simulink subsystem "Segway"  (R2023a)
settings: Solver=VariableStepAuto  StartTime=0.0  StopTime=10.0  RelTol=1e-3
settings Model: Creator=mfilo  LastModifiedBy=mfilo

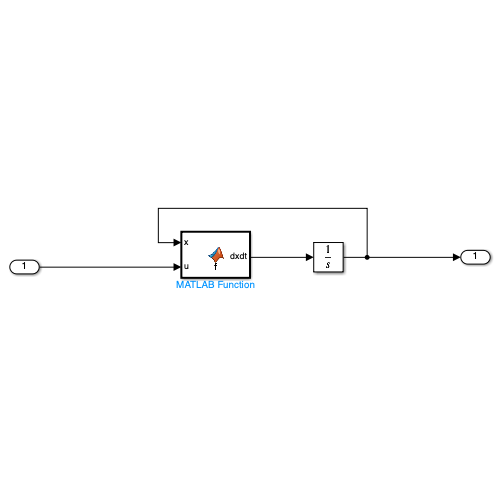
[thumbnail: Simulink's stored preview of the top-level diagram]
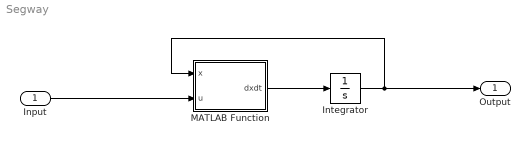
== system Segway ==
  Input : Inport
  Integrator : Integrator  InitialCondition=zeros(6,1)
  MATLAB Function : MATLAB Function  TreatAsAtomicUnit=on
  Output : Outport
  wires:
  Input/1 -> MATLAB Function/2(u)
  MATLAB Function/1(dxdt) -> Integrator/1
  Integrator/1 -> Output/1, MATLAB Function/1(x)

== matlab function Segway/MATLAB Function ==
  data: x input; u input; dxdt output
function dxdt = f(x, u)
    %% Parameters
    m = 0.141;      % [kg]
    M = 2.313;      % [kg]
    h = 0.254;      % [m]
    a = 0.165;      % [m]
    r = 0.0615;     % [m]
    I = 2.5e-4;     % [kg.m^2]
    I_x = 0.1986;   % [kg.m^2]
    I_y = 0.1942;   % [kg.m^2]
    I_z = 0.0056;   % [kg.m^2]]
    g = 9.81;       % [N.m^2/kg^2]

    %% Inputs
    T_l = u(1);
    T_r = u(2);

    %% States
    rho = x(1);
    psi = x(2);
    theta = x(3);
    v = x(4);
    omega_1 = x(5);
    omega_2 = x(6);

    %% Function
    dxdt = [v; ...
            omega_1; ...
            omega_2; ...
            (r^2*(M*h^2 + I_y)*(M*h*r*sin(theta)*omega_1^2 + M*h*r*sin(theta)*omega_2^2 + T_l + T_r))/(M^2*h^2*r^3*sin(theta)^2 + 2*m*M*h^2*r^3 + 2*I*M*h^2*r + I_y*M*r^3 + 2*I_y*m*r^3 + 2*I*I_y*r) + (M*h*r^2*cos(theta)*(- cos(theta)*sin(theta)*(M*h^2 + I_x - I_z)*omega_1^2 + T_l + T_r - M*g*h*sin(theta)))/(- M^2*h^2*r^2*cos(theta)^2 + M^2*h^2*r^2 + 2*m*M*h^2*r^2 + 2*I*M*h^2 + I_y*M*r^2 + 2*I_y*m*r^2 + 2*I*I_y); ...
           -(r^2*((a*(T_l - T_r))/r + omega_1*omega_2*cos(theta)*sin(theta)*(2*m*h^2 + 2*I_x - 2*I_z) + M*h*omega_1*v*sin(theta)))/(2*m*a^2*r^2 + 2*I*a^2 + M*h^2*r^2*sin(theta)^2 + I_z*r^2*cos(theta)^2 + I_x*r^2*sin(theta)^2); ...
           -((2*I + M*r^2 + 2*m*r^2)*(- cos(theta)*sin(theta)*(M*h^2 + I_x - I_z)*omega_1^2 + T_l + T_r - M*g*h*sin(theta)))/(- M^2*h^2*r^2*cos(theta)^2 + M^2*h^2*r^2 + 2*m*M*h^2*r^2 + 2*I*M*h^2 + I_y*M*r^2 + 2*I_y*m*r^2 + 2*I*I_y) - (M*h*r^2*cos(theta)*((T_l + T_r)/r + M*h*sin(theta)*(omega_1^2 + omega_2^2)))/(- M^2*h^2*r^2*cos(theta)^2 + M^2*h^2*r^2 + 2*m*M*h^2*r^2 + 2*I*M*h^2 + I_y*M*r^2 + 2*I_y*m*r^2 + 2*I*I_y)];
end
